simulink model "hello_world_2012b"  (R2012b)
settings: Solver=ode45  StartTime=0.0  StopTime=inf  RelTol=1e-3
libraries: dspnetwork x2
settings Model: Creator=Rishabh  LastModifiedBy=CCRE
settings DataIOCC: SaveFormat=StructureWithTime
settings OptimizationCC: ExpressionDepthLimit=128
settings DebuggingCC: UnderspecifiedInitializationDetection=Simplified  MergeDetectMultiDrivingBlocksExec=error  SolverPrmCheckMsg=none  FrameProcessingCompatibilityMsg=error  StateNameClashWarn=none
settings HardwareCC: ProdBitPerPointer=64  ProdLargestAtomicFloat=Float  ProdIntDivRoundTo=Zero  ProdEndianess=LittleEndian  ProdHWDeviceType=Specified
settings CodeAppCC: CustomSymbolStrType=$N$R$M_T
settings GRTTargetCC: CodeReplacementLibrary=C89/C90 (ANSI)  GeneratePreprocessorConditionals=Use local settings

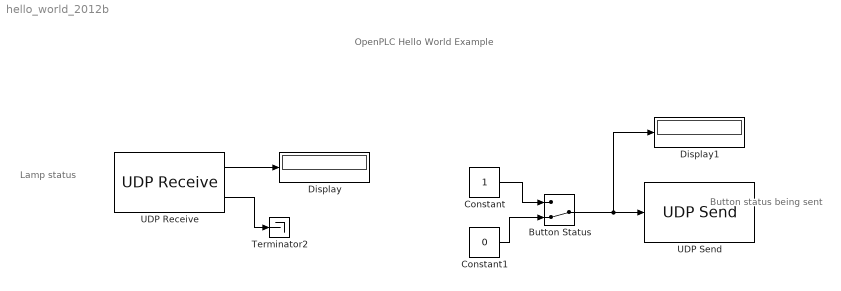
== system hello_world_2012b ==
  note: OpenPLC Hello World Example
  note: Lamp status
  note: Button status being sent
  Button Status : ManualSwitch  CurrentSetting=0
  Constant : Constant
  Constant1 : Constant  Value=0
  Display : Display
  Display1 : Display
  Terminator2 : Terminator
  UDP Receive : dspnetwork/UDP Receive  localURL='0.0.0.0'  localPort=10002  remoteURL='0.0.0.0'  remotePort=-1  recvBufferSize=2  dims=1  signalDatatype=uint16  isVarSize=off  showBlockingTime=on  blockingTime=0  sampletime=0.1  blockPlatform=LINUX
  UDP Send : dspnetwork/UDP Send  remoteURL='localhost'  remotePort=10001  localURL='255.255.255.255'  localPortSource=Automatically determine  localPort=-1  sampletime=-1  blockPlatform=LINUX  separateLengthPort=0
  wires:
  UDP Receive/2 -> Terminator2/1
  UDP Receive/1 -> Display/1
  Button Status/1 -> Display1/1, UDP Send/1
  Constant/1 -> Button Status/1
  Constant1/1 -> Button Status/2
